simulink subsystem "ApplFOCSLSysControl"  (R2024b)
settings: Solver=VariableStepAuto  StartTime=0.0  StopTime=10.0  RelTol=1e-3
values from neighbouring files (symbols this model uses):
  Ts = 2 * T_pwm    (= 0.0001)    [s32k344Data.m]
  Ts_speed = 20*Ts    [mcbSensorlessData.m]
undefined symbols (not defined in the file or in its folder): inverter, Per, pmsm, Unit
libraries: mcbcontrollergainlib x1
settings Model: Creator=The MathWorks, Inc.  LastModifiedBy=snarayan
settings RTWCC: GPUComputeCapability=3.5  LargeConstantGeneration=WriteOnlyDNNConstantsToDataFiles

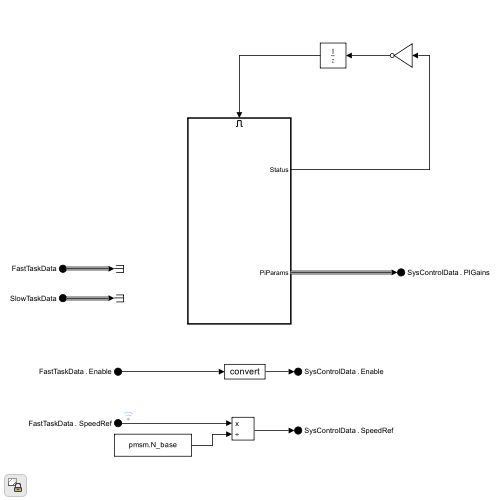
[thumbnail: Simulink's stored preview of the top-level diagram]
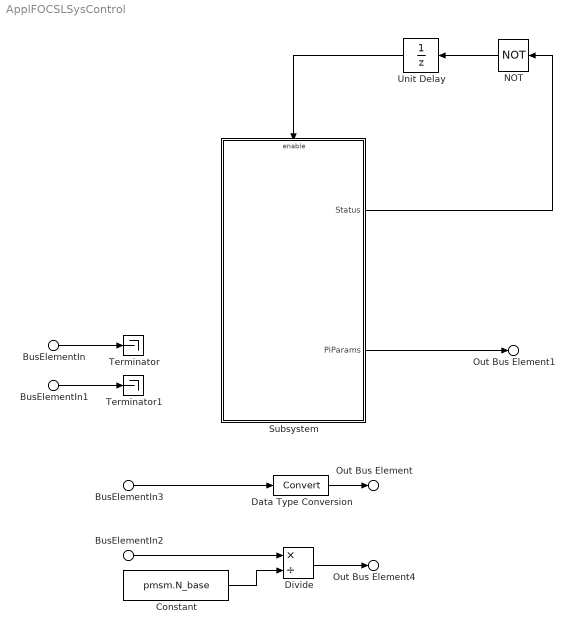
== system ApplFOCSLSysControl ==
  BusElementIn : Inport  PortName=FastTaskData
  BusElementIn2 : Inport  PortName=FastTaskData  Element=SpeedRef
  BusElementIn3 : Inport  PortName=FastTaskData  Element=Enable
  BusElementIn1 : Inport  Port=2  PortName=SlowTaskData
  Constant : Constant  Value=pmsm.N_base  OutDataTypeStr=dataType
  Data Type Conversion : DataTypeConversion  SaturateOnIntegerOverflow=off  RndMeth=Floor
  Divide : Product  Inputs=*/  RndMeth=Simplest  OutDataTypeStr=Inherit: Same as first input
  NOT : Logic  Operator=NOT  IconShape=distinctive  AllPortsSameDT=off  OutDataTypeStr=boolean
  Subsystem : Subsystem
  Terminator : Terminator
  Terminator1 : Terminator
  Unit Delay : UnitDelay  SampleTime=-1  HasFrameUpgradeWarning=on
  Out Bus Element : Outport  PortName=SysControlData  Element=Enable
  Out Bus Element1 : Outport  PortName=SysControlData  Element=PIGains
  Out Bus Element4 : Outport  PortName=SysControlData  Element=SpeedRef
  wires:
  BusElementIn1/1 -> Terminator1/1
  BusElementIn/1 -> Terminator/1
  Subsystem/2(PiParams) -> Out Bus Element1/1
  NOT/1 -> Unit Delay/1
  Subsystem/1(Status) -> NOT/1
  Unit Delay/1 -> Subsystem/Enable
  Data Type Conversion/1 -> Out Bus Element/1
  Constant/1 -> Divide/2
  BusElementIn3/1 -> Data Type Conversion/1
  Divide/1 -> Out Bus Element4/1
  BusElementIn2/1 -> Divide/1

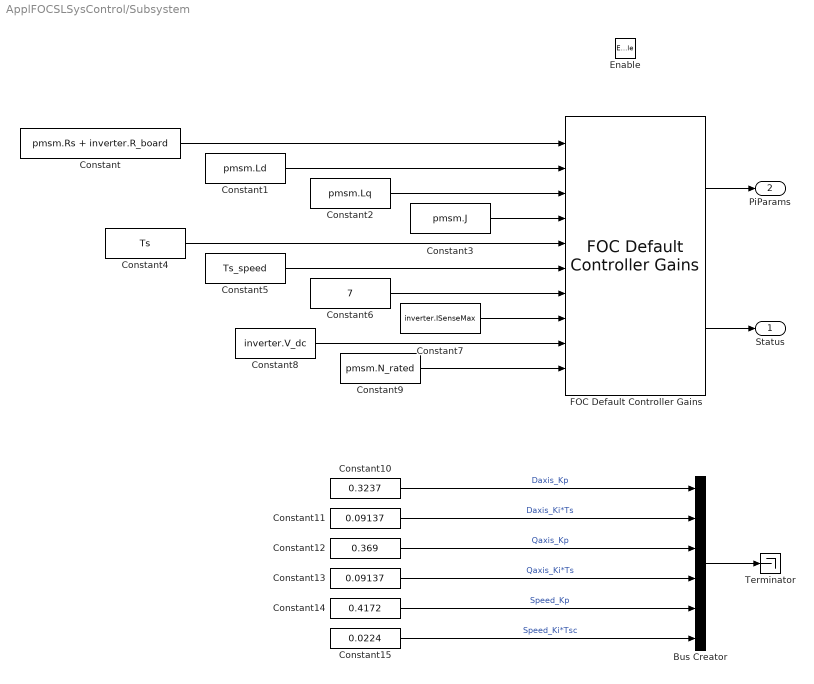
== system ApplFOCSLSysControl/Subsystem ==
  Enable : EnablePort
  Bus Creator : BusCreator  Inputs=6
  Constant : Constant  Value=pmsm.Rs + inverter.R_board  OutDataTypeStr=dataType
  Constant1 : Constant  Value=pmsm.Ld  OutDataTypeStr=dataType
  Constant10 : Constant  Value=0.3237  OutDataTypeStr=dataType
  Constant11 : Constant  Value=0.09137  OutDataTypeStr=dataType
  Constant12 : Constant  Value=0.369  OutDataTypeStr=dataType
  Constant13 : Constant  Value=0.09137  OutDataTypeStr=dataType
  Constant14 : Constant  Value=0.4172  OutDataTypeStr=dataType
  Constant15 : Constant  Value=0.0224  OutDataTypeStr=dataType
  Constant2 : Constant  Value=pmsm.Lq  OutDataTypeStr=dataType
  Constant3 : Constant  Value=pmsm.J  OutDataTypeStr=dataType
  Constant4 : Constant  Value=Ts  OutDataTypeStr=dataType
  Constant5 : Constant  Value=Ts_speed  OutDataTypeStr=dataType
  Constant6 : Constant  Value=7  OutDataTypeStr=dataType
  Constant7 : Constant  Value=inverter.ISenseMax  OutDataTypeStr=dataType
  Constant8 : Constant  Value=inverter.V_dc  OutDataTypeStr=dataType
  Constant9 : Constant  Value=pmsm.N_rated  OutDataTypeStr=dataType
  FOC Default Controller Gains : mcbcontrollergainlib/FOC Default Controller Gains  motorSelection=PMSM  unitType=Per-Unit  outCurrentControlGain=on  outFWCGain=off  outSpeedControlGain=on  externalDelay=off  currentSensorDelay=50e-6  speedSensorDelay=50e-6  speedFilterDelay=0.02
  Terminator : Terminator
  Status : Outport
  PiParams : Outport  Port=2
  wires:
  Bus Creator/1 -> Terminator/1
  FOC Default Controller Gains/1 -> PiParams/1
  Constant15/1 -> Bus Creator/6  "Speed_Ki*Tsc"
  Constant14/1 -> Bus Creator/5  "Speed_Kp"
  Constant13/1 -> Bus Creator/4  "Qaxis_Ki*Ts"
  Constant12/1 -> Bus Creator/3  "Qaxis_Kp"
  Constant11/1 -> Bus Creator/2  "Daxis_Ki*Ts"
  Constant10/1 -> Bus Creator/1  "Daxis_Kp"
  Constant/1 -> FOC Default Controller Gains/1
  FOC Default Controller Gains/2 -> Status/1
  Constant8/1 -> FOC Default Controller Gains/9
  Constant6/1 -> FOC Default Controller Gains/7
  Constant7/1 -> FOC Default Controller Gains/8
  Constant2/1 -> FOC Default Controller Gains/3
  Constant4/1 -> FOC Default Controller Gains/5
  Constant3/1 -> FOC Default Controller Gains/4
  Constant9/1 -> FOC Default Controller Gains/10
  Constant5/1 -> FOC Default Controller Gains/6
  Constant1/1 -> FOC Default Controller Gains/2
